simulink model "CCCV"  (R2019a)
settings: Solver=VariableStepAuto  StartTime=0.0  StopTime=50000  RelTol=1e-3
undefined symbols (not defined in the file or in its folder): Ion, Lithium
libraries: powerlib x13, electricdrivelib x1
settings Model: SimulationMode=accelerator  Creator=kagom  LastModifiedBy=kagom
settings SolverCC: ZeroCrossAlgorithm=Adaptive
settings DebuggingCC: IgnoredZcDiagnostic=none

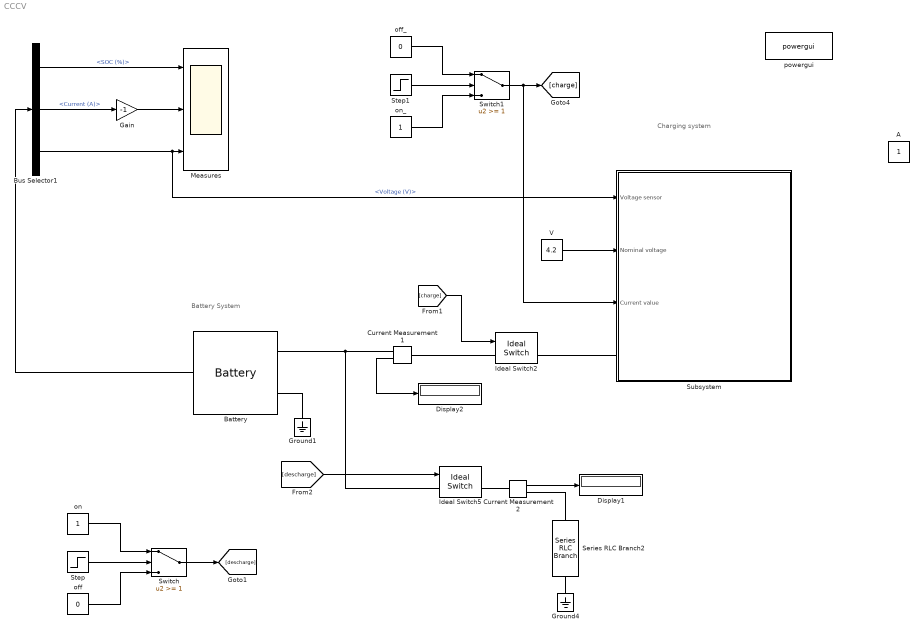
== system CCCV ==
  note: Battery System
  note: Charging system
  A : Constant
  Battery : electricdrivelib/Extra Sources/Battery  BatType=Lithium-Ion  ShowTempParam=off  ThermalPreset=no  ShowAgeParam=off  NomV=3.7  NomQ=3.3  SOC=0  Batt_Tr=30  PresetModel=on  MaxQ=3.3  MinV=2.775  FullV=4.3068  Dis_rate=1.4348  R=0.011212  Normal_OP=2.9843  expZone="[3.9974     0.16213]"  current=[6.5 13 32.5]  Units=Time  Tci=25  NomT=25  T2=0  MaxQ2=2.208  FullV2=3.45  Normal_OP2=2.8  expZone2="[3.22        0.23]"  Rca=0.6  ti=1000  Dp=0  Neq0=0  Tsim=1e6  Ta1=25  Qeol=5.4*0.9  Reol=0.013333*1.2  Char_age=[2.3478, 3]  Dis_age=[2.3478, 10]  N1=1500  N2=10500  N3=1000  N4=1400  Ta2=45  N5=950
      settings: SourceProductName=Simscape Electrical
  Bus Selector1 : BusSelector  OutputSignals=SOC (%),Current (A),Voltage (V)
  Current Measurement1 : powerlib/Measurements/Current Measurement  PhasorSimulation=off  OutputType=Complex  PSBequivalent=0
      settings: SourceProductName=Simscape Electrical
  Current Measurement2 : powerlib/Measurements/Current Measurement  PhasorSimulation=off  OutputType=Complex  PSBequivalent=0
      settings: SourceProductName=Simscape Electrical
  Display1 : Display
  Display2 : Display
  Gain : Gain  Gain=-1
  Ground1 : powerlib/Elements/Ground  LConnTagsString=a
      settings: SourceProductName=Simscape Electrical
  Ground4 : powerlib/Elements/Ground  LConnTagsString=a
      settings: SourceProductName=Simscape Electrical
  Ideal Switch2 : powerlib/Power Electronics/Ideal Switch  Ron=0.001  Lon=0  IC=0  Rs=1e5  Cs=inf  Measurements=on
      settings: SourceProductName=Simscape Electrical
  Ideal Switch5 : powerlib/Power Electronics/Ideal Switch  Ron=0.001  Lon=0  IC=0  Rs=1e5  Cs=inf  Measurements=on
      settings: SourceProductName=Simscape Electrical
  "Measures " : Scope  NumInputPorts=3
  Series RLC Branch2 : powerlib/Elements/Series RLC Branch  LConnTagsString=__new0  RConnTagsString=__new0  BranchType=R  Resistance=10  Inductance=1e-3  SetiL0=off  InitialCurrent=0  Capacitance=1e-6  Setx0=off  InitialVoltage=0  Measurements=None
      settings: SourceProductName=Simscape Electrical
  Step : Step  Time=12922.8  SampleTime=0
  Step1 : Step  Time=12922.8  SampleTime=0
  Subsystem : Subsystem
      settings: AttributesFormatString=MCU_S1
  Switch : Switch  Threshold=1
  Switch1 : Switch  Threshold=1
  V : Constant  Value=4.2
  off : Constant  Value=0
  off_ : Constant  Value=0
  on : Constant
  on_ : Constant
  powergui : powerlib/powergui  SimulationMode=Continuous  SampleTime=0.001  frequency=60  Iterations=50  frequencyindice=0  Pbase=100e6  ErrMax=1e-4  UnitsV=kV  UnitsW=MW  buscounter=0  FunctionMessages=off  echomessages=off  EnableUseOfTLC=off  CurrentSourceSwitches=off  DisableSnubberDevices=off  DisableRonSwitches=off  DisableVfSwitches=off  DisplayEquations=off  AutomaticDiscreteSolvers=off  SolverType=Tustin  Interpol=off  ExternalGateDelay=off  methode=off  Ts=0  x0status=blocks  SPID=on  SwTol=0  HookPort=off  NonlinearTolerance=0  nMaxIteration=15  ContinueOnMaxIteration=off  RestoreLinks=warning  ResistiveCurrentMeasurement=off  Frange=[0:2:500]  Ylog=off  Xlog=on  ShowGrid=off  save=off  variable=ZData  structure=0  ZoomFFT=on  StartTime=0.0  cycles=1  DisplayStyle=1  fundamental=60  FreqAxis=off  MaxFrequency=1000  frequencyindicesteady=1  RmsSteady=1  display=off
      settings: SourceProductName=Simscape Electrical
  wires:
  Bus Selector1/2 -> Gain/1  "<Current (A)>"
  Current Measurement2/1 -> Display1/1
  V/1 -> Subsystem/2(Nominal voltage)
  Bus Selector1/3 -> Subsystem/1(Voltage sensor), "Measures "/3  "<Voltage (V)>"
  Gain/1 -> "Measures "/2
  Battery/1 -> Bus Selector1/1
  Bus Selector1/1 -> "Measures "/1  "<SOC (%)>"
  off/1 -> Switch/3
  on/1 -> Switch/1
  Step/1 -> Switch/2
  on_/1 -> Switch1/3
  off_/1 -> Switch1/1
  Step1/1 -> Switch1/2
  [charge] -> Ideal Switch2/1
  [descharge] -> Ideal Switch5/1
  Switch1/1 -> Subsystem/3(Current value), [charge]
  Switch/1 -> [descharge]
  Current Measurement1/1 -> Display2/1
  connections:
  Ground1/LConn1 -- Battery/LConn2
  Ideal Switch5/LConn1 -- Battery/LConn1 -- Current Measurement1/RConn1
  Current Measurement2/RConn1 -- Series RLC Branch2/LConn1
  Ground4/LConn1 -- Series RLC Branch2/RConn1
  Ideal Switch5/RConn1 -- Current Measurement2/LConn1
  Ideal Switch2/RConn1 -- Subsystem/LConn1
  Current Measurement1/LConn1 -- Ideal Switch2/LConn1

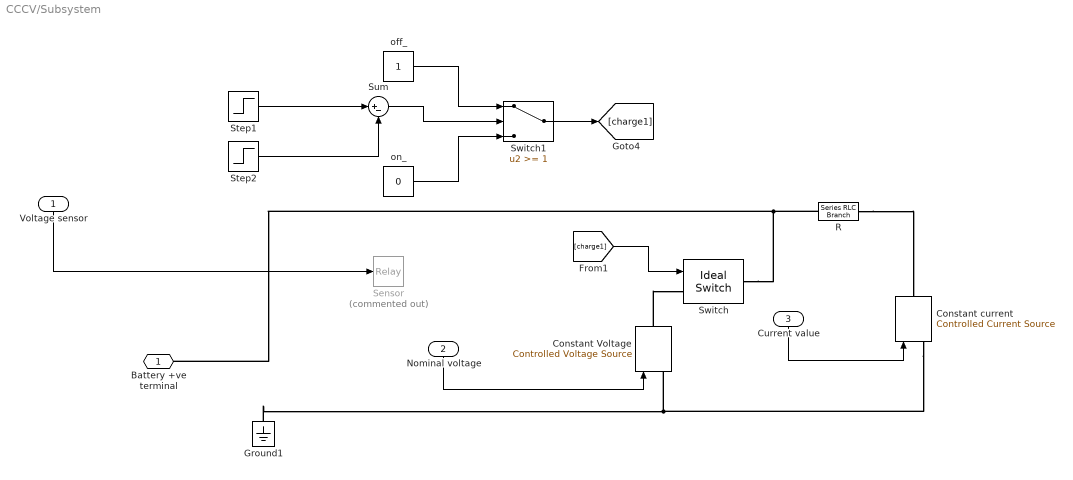
== system CCCV/Subsystem ==
  Voltage sensor : Inport
  Nominal voltage : Inport  Port=2
  Current value : Inport  Port=3
  Constant Voltage : powerlib/Electrical Sources/Controlled Voltage Source  Initialize=on  Source_Type=DC  Amplitude=0  Phase=0  Frequency=0  Measurements=None
      settings: SourceProductName=Simscape Electrical
  "Constant current " : powerlib/Electrical Sources/Controlled Current Source  Initialize=on  Source_Type=DC  Amplitude=0  Phase=0  Frequency=0  Measurements=None
      settings: SourceProductName=Simscape Electrical
  Ground1 : powerlib/Elements/Ground  LConnTagsString=a
      settings: SourceProductName=Simscape Electrical
  R : powerlib/Elements/Series RLC Branch  LConnTagsString=__new0  RConnTagsString=__new0  BranchType=R  Resistance=1000  Inductance=0  SetiL0=off  InitialCurrent=0  Capacitance=0  Setx0=off  InitialVoltage=0  Measurements=Branch voltage
      settings: SourceProductName=Simscape Electrical
  Sensor : Relay  Commented=on  OnSwitchValue=4.2  OffSwitchValue=4.2
  Step1 : Step  Time=11670.75  SampleTime=0
  Step2 : Step  Time=12922.8  SampleTime=0
  Sum : Sum  Inputs=|+-
  Switch : powerlib/Power Electronics/Ideal Switch  Ron=0  Lon=0  IC=0  Rs=1e5  Cs=inf  Measurements=off
      settings: SourceProductName=Simscape Electrical
  Switch1 : Switch  Threshold=1
  off_ : Constant
  on_ : Constant  Value=0
  Battery +ve terminal : PMIOPort  Side=Left
  wires:
  Nominal voltage/1 -> Constant Voltage/1
  Current value/1 -> "Constant current "/1
  Voltage sensor/1 -> Sensor/1
  Switch1/1 -> [charge1]
  off_/1 -> Switch1/1
  on_/1 -> Switch1/3
  Step1/1 -> Sum/1
  Sum/1 -> Switch1/2
  Step2/1 -> Sum/2
  [charge1] -> Switch/1
  connections:
  "Constant current "/LConn1 -- Ground1/LConn1 -- Constant Voltage/LConn1
  R/LConn1 -- Battery +ve terminal/RConn1 -- Switch/RConn1
  R/RConn1 -- "Constant current "/RConn1
  Constant Voltage/RConn1 -- Switch/LConn1
